simulink model "a6_2_solving_high_level_equations"  (R2018a)
settings: Solver=VariableStepAuto  StartTime=0.0  StopTime=10.0  RelTol=1e-3
settings Model: Creator=r0x6f736f646f  LastModifiedBy=r0x6f736f646f

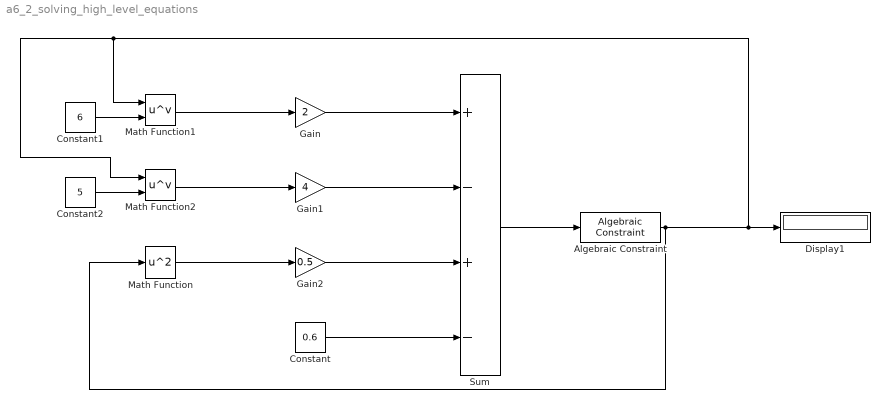
== system a6_2_solving_high_level_equations ==
  Algebraic Constraint : AlgebraicConstraint
  Constant : Constant  Value=0.6
  Constant1 : Constant  Value=6
  Constant2 : Constant  Value=5
  Display1 : Display
  Gain : Gain  Gain=2
  Gain1 : Gain  Gain=4
  Gain2 : Gain  Gain=0.5
  Math Function : Math  Operator=square  SaturateOnIntegerOverflow=on
  Math Function1 : Math  Operator=pow  SaturateOnIntegerOverflow=on
  Math Function2 : Math  Operator=pow  SaturateOnIntegerOverflow=on
  Sum : Sum  Inputs=+-+-
  wires:
  Sum/1 -> Algebraic Constraint/1
  Gain/1 -> Sum/1
  Math Function1/1 -> Gain/1
  Gain1/1 -> Sum/2
  Gain2/1 -> Sum/3
  Constant/1 -> Sum/4
  Math Function2/1 -> Gain1/1
  Math Function/1 -> Gain2/1
  Constant2/1 -> Math Function2/2
  Constant1/1 -> Math Function1/2
  Algebraic Constraint/1 -> Math Function/1, Math Function2/1, Math Function1/1, Display1/1
